simulink model "chuaTracking_sim"  (R2024a)
settings: Solver=VariableStepAuto  StartTime=0.0  StopTime=t_sim  RelTol=1e-3
values from neighbouring files (symbols this model uses):
  K = place(A, B, l_des)    [ChuaFL.m]    (also in chuaFLUnexact.m)
settings Model: Creator=lorenzo  LastModifiedBy=lorenzo

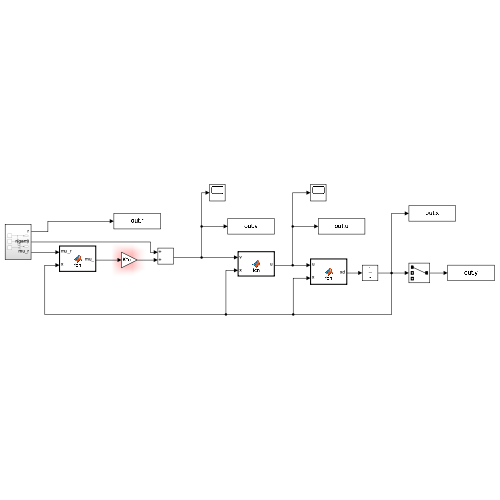
[thumbnail: Simulink's stored preview of the top-level diagram]
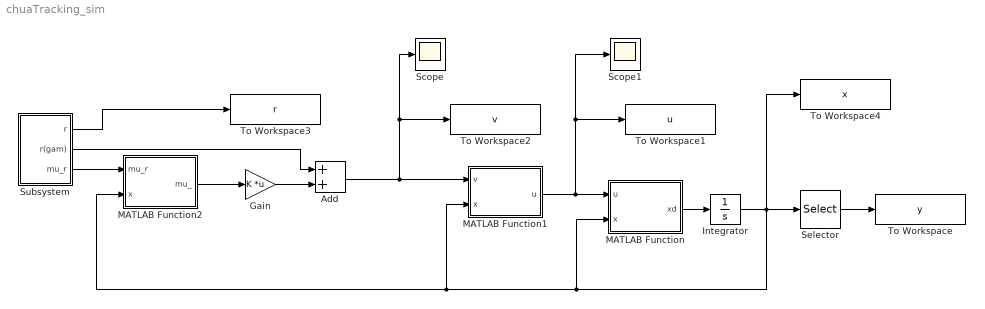
== system chuaTracking_sim ==
  Add : Sum
  Gain : Gain  Gain=K  Multiplication=Matrix(K*u)
  Integrator : Integrator
  MATLAB Function : MATLAB Function  TreatAsAtomicUnit=on
  MATLAB Function1 : MATLAB Function  TreatAsAtomicUnit=on
  MATLAB Function2 : MATLAB Function  TreatAsAtomicUnit=on
  Scope : Scope
  Scope1 : Scope
  Selector : Selector  InputPortWidth=3  IndexOptions=Index vector (dialog)  Indices=1  OutputSizes=1
  Subsystem : Subsystem
  To Workspace : ToWorkspace  VariableName=y  SaveFormat=Timeseries  SampleTime=-1
  To Workspace1 : ToWorkspace  VariableName=u  SaveFormat=Timeseries  SampleTime=-1
  To Workspace2 : ToWorkspace  VariableName=v  SaveFormat=Timeseries  SampleTime=-1
  To Workspace3 : ToWorkspace  VariableName=r  SaveFormat=Timeseries  SampleTime=-1
  To Workspace4 : ToWorkspace  VariableName=x  SaveFormat=Timeseries  SampleTime=-1
  wires:
  MATLAB Function/1(xd) -> Integrator/1
  Integrator/1 -> To Workspace4/1, MATLAB Function/2(x), MATLAB Function2/2(x), MATLAB Function1/2(x), Selector/1
  MATLAB Function1/1(u) -> To Workspace1/1, Scope1/1, MATLAB Function/1(u)
  Add/1 -> MATLAB Function1/1(v), Scope/1, To Workspace2/1
  Gain/1 -> Add/2
  Subsystem/3(mu_r) -> MATLAB Function2/1(mu_r)
  Subsystem/2(r(gam)) -> Add/1
  Subsystem/1(r) -> To Workspace3/1
  Selector/1 -> To Workspace/1
  MATLAB Function2/1(mu_) -> Gain/1

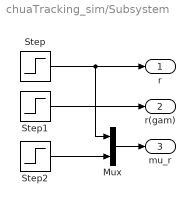
== system chuaTracking_sim/Subsystem ==
  Mux : Mux  Inputs=2
  Step : Step  Time=0  SampleTime=0
  Step1 : Step  Time=0  After=0  SampleTime=0
  Step2 : Step  Time=0  After=0  SampleTime=0
  r : Outport  VectorParamsAs1DForOutWhenUnconnected=off
  r(gam) : Outport  Port=2  VectorParamsAs1DForOutWhenUnconnected=off
  mu_r : Outport  Port=3  VectorParamsAs1DForOutWhenUnconnected=off
  wires:
  Step/1 -> Mux/1, r/1
  Step1/1 -> r(gam)/1
  Step2/1 -> Mux/2
  Mux/1 -> mu_r/1

== matlab function chuaTracking_sim/MATLAB Function1 ==
  data: v input; u output; x input
function u = fcn(v,x)

alpha = 10.4;
rho = -1.16*x(1) + 0.041*x(1)^3;
rhod = (123*x(1)^2)/1000 - 29/25;

u = v/alpha - (x(1)-x(2)+x(3)-alpha*(x(2)-x(1)-rho)*(1+rhod));

== matlab function chuaTracking_sim/MATLAB Function ==
  data: u input; xd output; x input
function xd = fcn(u,x)

R = 0.1; alpha = 10.4; beta = 16.5;
rho = -1.16*x(1) + 0.041*x(1)^3;

xd = [alpha*(x(2)-x(1)-rho);
 x(1)-x(2)+x(3)+u;
 -beta*x(2)-R*x(3)];

== matlab function chuaTracking_sim/MATLAB Function2 ==
  data: mu_r input; x input; mu_ output
function mu_ = fcn(mu_r,x)

alpha = 10.4;
rho = -1.16*x(1) + 0.041*x(1)^3;
mu = [x(1); alpha*(x(2)-x(1)-rho)];

mu_ = mu_r - mu;
